simulink model "ysw11_18"  (R2014a)
settings: Solver=ode45  StartTime=0.0  StopTime=10.0  RelTol=1e-3
libraries: commdigbbndfm2 x1
settings Model: Creator=ii  LastModifiedBy=ii
settings SolverCC: ZeroCrossAlgorithm=Adaptive
settings DebuggingCC: UnderspecifiedInitializationDetection=Classic

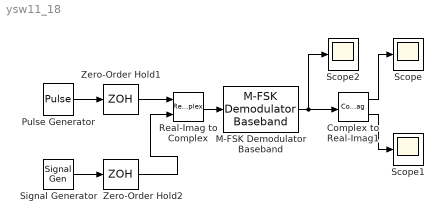
== system ysw11_18 ==
  Complex to Real-Imag1 : ComplexToRealImag
  M-FSK Demodulator Baseband : commdigbbndfm2/M-FSK Demodulator Baseband  M=32  OutType=Bit  Dec=Gray  freqSep=1  numSamp=2  RateOptions=Inherit from input (this choice will be removed - see release notes)  outDataType=double
  Pulse Generator : DiscretePulseGenerator  PulseType=Time based  Amplitude=300  Period=10  PulseWidth=5
  Real-Imag to Complex : RealImagToComplex
  Scope : Scope
  Scope1 : Scope
  Scope2 : Scope
      settings: SaveName=ScopeData2
  Signal Generator : SignalGenerator  Amplitude=100  Frequency=1000  Units=rad/sec
  Zero-Order Hold1 : ZeroOrderHold
  Zero-Order Hold2 : ZeroOrderHold
  wires:
  M-FSK Demodulator Baseband/1 -> Scope2/1, Complex to Real-Imag1/1
  Complex to Real-Imag1/1 -> Scope/1
  Complex to Real-Imag1/2 -> Scope1/1
  Zero-Order Hold1/1 -> Real-Imag to Complex/1
  Pulse Generator/1 -> Zero-Order Hold1/1
  Signal Generator/1 -> Zero-Order Hold2/1
  Zero-Order Hold2/1 -> Real-Imag to Complex/2
  Real-Imag to Complex/1 -> M-FSK Demodulator Baseband/1
